simulink model "MPC_simulink"  (R2019b)
settings: Solver=VariableStepAuto  StartTime=0.0  StopTime=inf  RelTol=1e-3
InitFcn:
  | setup_NMPC
undefined symbols (not defined in the file or in its folder): MPC_func
libraries: modbusMatLib x12, simulink x7, dspstat3 x3, realtime_pacer_lib x1
settings Model: Creator=pppc  LastModifiedBy=Lenovo
settings SFSimCC: CustomCodeUndefinedFunction=UseInterfaceOnly

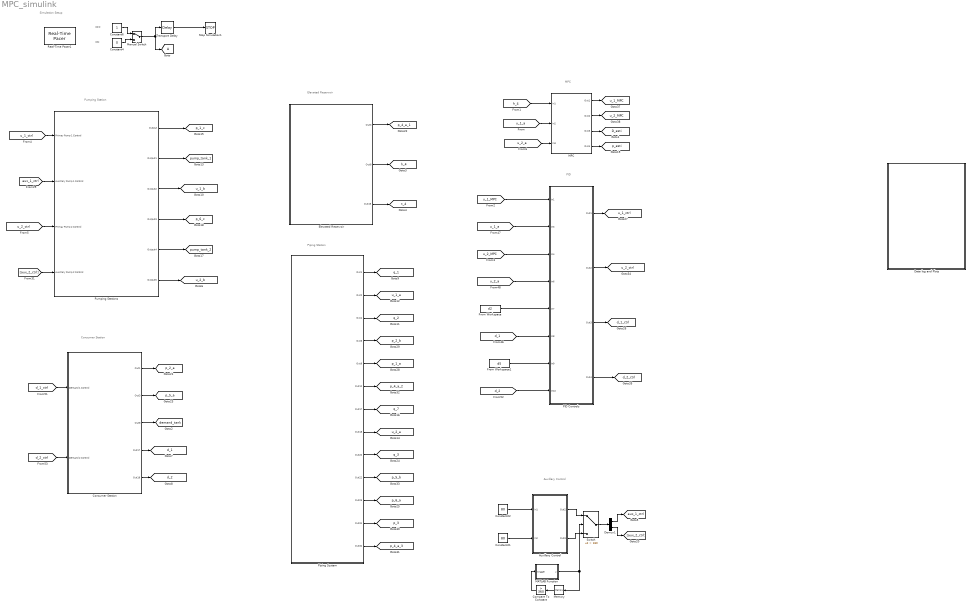
== system MPC_simulink ==
  note: Pumping Station
  note: ON
  note: Simulation Setup
  note: OFF
  note: Consumer Station
  note: Elevated Reservoir
  note: Piping Station
  note: MPC
  note: PID
  note: Auxillary Control
  Auxillary Control : Subsystem
  Compare To Constant : simulink/Logic and Bit Operations/Compare To Constant  relop=>  const=360  OutDataTypeStr=uint8
  Constant21 : Constant  Value=80
  Constant22 : Constant  Value=80
  Constant4 : Constant  Value=0
  Constant6 : Constant
  Consumer Station : Subsystem
  Data log and Plots : Subsystem
  Demux1 : Demux  Outputs=2
  "Elevated Reservoir " : Subsystem
  From Workspace : FromWorkspace  VariableName=d2  SampleTime=1
  From Workspace1 : FromWorkspace  VariableName=d5  SampleTime=1
  MATLAB Function : MATLAB Function  TreatAsAtomicUnit=on  SystemSampleTime=1
  MPC : Subsystem
  Manual Switch : ManualSwitch
  Memory : Memory
  "PID Controls " : Subsystem
  Piping System : Subsystem
  Pumping Stations : Subsystem
  Real-Time Pacer1 : realtime_pacer_lib/Real-Time Pacer  simTimePerRealTime=1
  Stop Simulation1 : Stop
  Switch : Switch  Criteria=u2 > Threshold  Threshold=180
  Transport Delay : TransportDelay  DelayTime=2
  tag scope: A=global, D_esti=global, aux_1_ctrl=global, d_1=global, d_1_ctrl=global, d_2=global, d_2_ctrl=global, demand_tank=global, h_4=global, p_1_a=global, p_1_c=global, p_2_a=global, p_2_b=global, p_3=global, p_4_a_1=global, p_4_a_2=global, p_4_a_3=global, p_5_a=global, p_5_b=global, p_6_a=global, p_6_c=global, p_esti=global, pump_tank_1=global, pump_tank_2=global, q_1=global, q_2=global, q_3=global, q_7=global, t_4=global, u_1_MPC=global, u_1_a=global, u_1_b=global, u_1_ctrl=global, u_2_MPC=global, u_2_a=global, u_2_b=global, u_2_ctrl=global
  wires:
  Manual Switch/1 -> [A], Transport Delay/1
  Constant4/1 -> Manual Switch/2
  Transport Delay/1 -> Stop Simulation1/1
  Constant6/1 -> Manual Switch/1
  [u_1_ctrl] -> Pumping Stations/1(Primay Pump 1 Control)
  [u_2_ctrl] -> Pumping Stations/3(Primay Pump 2 Control)
  [aux_2_ctrl] -> Pumping Stations/4(Auxillary Pump 2 Control)
  [aux_1_ctrl] -> Pumping Stations/2(Auxillary Pump 1 Control)
  Pumping Stations/1(Output) -> [p_1_c]
  Pumping Stations/2(Output1) -> [pump_tank_1]
  Pumping Stations/3(Output2) -> [u_1_b]
  Pumping Stations/6(Output5) -> [u_2_b]
  Pumping Stations/5(Output4) -> [pump_tank_2]
  Pumping Stations/4(Output3) -> [p_6_c]
  [d_1_ctrl] -> Consumer Station/1(Demand 1 Control)
  [d_2_ctrl] -> Consumer Station/2(Demand 2 Control)
  Consumer Station/1(Out1) -> [p_2_a]
  Consumer Station/2(Out3) -> [p_5_a]
  Consumer Station/3(Out8) -> [demand_tank]
  Consumer Station/4(Out17) -> [d_1]
  Consumer Station/5(Out19) -> [d_2]
  "Elevated Reservoir "/1(Out3) -> [p_4_a_1]
  "Elevated Reservoir "/2(Out8) -> [h_4]
  "Elevated Reservoir "/3(Out19) -> [t_4]
  Piping System/1(Out1) -> [q_1]
  Piping System/2(Out2) -> [u_1_a]
  Piping System/3(Out4) -> [q_2]
  Piping System/4(Out6) -> [p_2_b]
  Piping System/5(Out9) -> [p_1_a]
  Piping System/6(Out12) -> [p_4_a_2]
  Piping System/7(Out17) -> [q_7]
  Piping System/8(Out18) -> [u_2_a]
  Piping System/9(Out20) -> [q_3]
  Piping System/10(Out22) -> [p_5_b]
  Piping System/11(Out25) -> [p_6_a]
  Piping System/12(Out31) -> [p_3]
  Piping System/13(Out32) -> [p_4_a_3]
  [u_1_MPC] -> "PID Controls "/1(In1)
  [u_1_a] -> "PID Controls "/2(In3)
  [u_2_MPC] -> "PID Controls "/3(In4)
  [u_2_a] -> "PID Controls "/4(In6)
  From Workspace/1 -> "PID Controls "/5(In7)
  [d_1] -> "PID Controls "/6(In8)
  From Workspace1/1 -> "PID Controls "/7(In9)
  [d_2] -> "PID Controls "/8(In10)
  "PID Controls "/1(Out1) -> [u_1_ctrl]
  "PID Controls "/2(Out2) -> [u_2_ctrl]
  "PID Controls "/3(Out3) -> [d_1_ctrl]
  "PID Controls "/4(Out4) -> [d_2_ctrl]
  [h_4] -> MPC/1(In1)
  MPC/1(Out1) -> [u_1_MPC]
  MPC/2(Out2) -> [u_2_MPC]
  Constant22/1 -> Auxillary Control/1(In1)
  Constant21/1 -> Auxillary Control/2(In2)
  Demux1/1 -> [aux_1_ctrl]
  Compare To Constant/1 -> MATLAB Function/1(trigger)
  Auxillary Control/2(Out3) -> Switch/3
  Switch/1 -> Demux1/1
  Auxillary Control/1(Out2) -> Switch/1
  Demux1/2 -> [aux_2_ctrl]
  MATLAB Function/1(y) -> Switch/2, Memory/1
  Memory/1 -> Compare To Constant/1
  MPC/3(Out3) -> [D_esti]
  MPC/4(Out4) -> [p_esti]
  [u_1_a] -> MPC/2(In2)
  [u_2_a] -> MPC/3(In3)

== system MPC_simulink/Auxillary Control ==
  In1 : Inport
  In2 : Inport  Port=2
  Auxillary control : MATLAB Function  TreatAsAtomicUnit=on
  Auxillary control1 : MATLAB Function  TreatAsAtomicUnit=on
  Constant23 : Constant  Value=0
  Mux1 : Mux  Inputs=2
  Mux2 : Mux  Inputs=2
  Out2 : Outport  VectorParamsAs1DForOutWhenUnconnected=off
  Out3 : Outport  Port=2  VectorParamsAs1DForOutWhenUnconnected=off
  wires:
  Constant23/1 -> Mux2/1, Mux1/2
  Auxillary control1/1(pumpsaux) -> Mux2/2
  [demand_tank] -> Auxillary control1/1(dp)
  In2/1 -> Auxillary control1/2(u_aux)
  [demand_tank] -> Auxillary control/1(dp)
  Mux2/1 -> Out3/1
  In1/1 -> Auxillary control/2(u_aux)
  Mux1/1 -> Out2/1
  Auxillary control/1(pumpsaux) -> Mux1/1

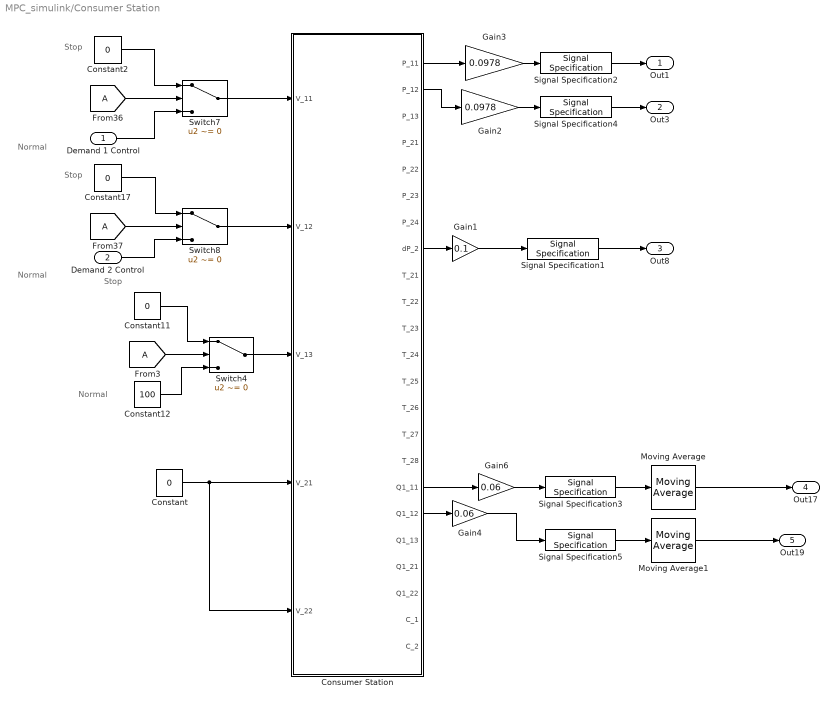
== system MPC_simulink/Consumer Station ==
  note: Normal
  note: Normal
  note: Stop
  note: Stop
  note: Normal
  note: Stop
  Demand 1 Control : Inport
  Demand 2 Control : Inport  Port=2
  Constant{,2,11,17} (4 alike) : Constant  Value=0
  Constant12 : Constant  Value=100
  Consumer Station : Subsystem
  Gain1 : Gain  Gain=0.1
  Gain2 : Gain  Gain=0.0978
  Gain3 : Gain  Gain=0.0978
  Gain4 : Gain  Gain=0.06
  Gain6 : Gain  Gain=0.06
  Moving Average : dspstat3/Moving Average  Method=Sliding window  ForgettingFactorPort=off  SpecifyWindowLength=on  WindowLength=13  ForgettingFactor=0.9  SimulateUsing=Code generation
  Moving Average1 : dspstat3/Moving Average  Method=Sliding window  ForgettingFactorPort=off  SpecifyWindowLength=on  WindowLength=13  ForgettingFactor=0.9  SimulateUsing=Code generation
  Signal Specification1 : SignalSpecification  Unit=m
  Signal Specification2 : SignalSpecification  Unit=bar
  Signal Specification3 : SignalSpecification  Unit=m^3/hr
  Signal Specification4 : SignalSpecification  Unit=bar
  Signal Specification5 : SignalSpecification  Unit=m^3/hr
  Switch4 : Switch  Criteria=u2 ~= 0
  Switch7 : Switch  Criteria=u2 ~= 0
  Switch8 : Switch  Criteria=u2 ~= 0
  Out1 : Outport  VectorParamsAs1DForOutWhenUnconnected=off
  Out3 : Outport  Port=2  VectorParamsAs1DForOutWhenUnconnected=off
  Out8 : Outport  Port=3  VectorParamsAs1DForOutWhenUnconnected=off
  Out17 : Outport  Port=4  VectorParamsAs1DForOutWhenUnconnected=off
  Out19 : Outport  Port=5  VectorParamsAs1DForOutWhenUnconnected=off
  wires:
  Constant11/1 -> Switch4/1
  Constant17/1 -> Switch8/1
  [A] -> Switch8/2
  Signal Specification1/1 -> Out8/1
  Constant12/1 -> Switch4/3
  Consumer Station/8(dP_2) -> Gain1/1
  Switch8/1 -> Consumer Station/2(V_12)
  Gain1/1 -> Signal Specification1/1
  Demand 2 Control/1 -> Switch8/3
  [A] -> Switch4/2
  Constant2/1 -> Switch7/1
  Switch4/1 -> Consumer Station/3(V_13)
  Signal Specification4/1 -> Out3/1
  Switch7/1 -> Consumer Station/1(V_11)
  Constant/1 -> Consumer Station/5(V_22), Consumer Station/4(V_21)
  [A] -> Switch7/2
  Demand 1 Control/1 -> Switch7/3
  Gain2/1 -> Signal Specification4/1
  Consumer Station/2(P_12) -> Gain2/1
  Gain3/1 -> Signal Specification2/1
  Signal Specification2/1 -> Out1/1
  Consumer Station/1(P_11) -> Gain3/1
  Signal Specification3/1 -> Moving Average/1
  Gain6/1 -> Signal Specification3/1
  Consumer Station/17(Q1_11) -> Gain6/1
  Gain4/1 -> Signal Specification5/1
  Consumer Station/18(Q1_12) -> Gain4/1
  Signal Specification5/1 -> Moving Average1/1
  Moving Average/1 -> Out17/1
  Moving Average1/1 -> Out19/1

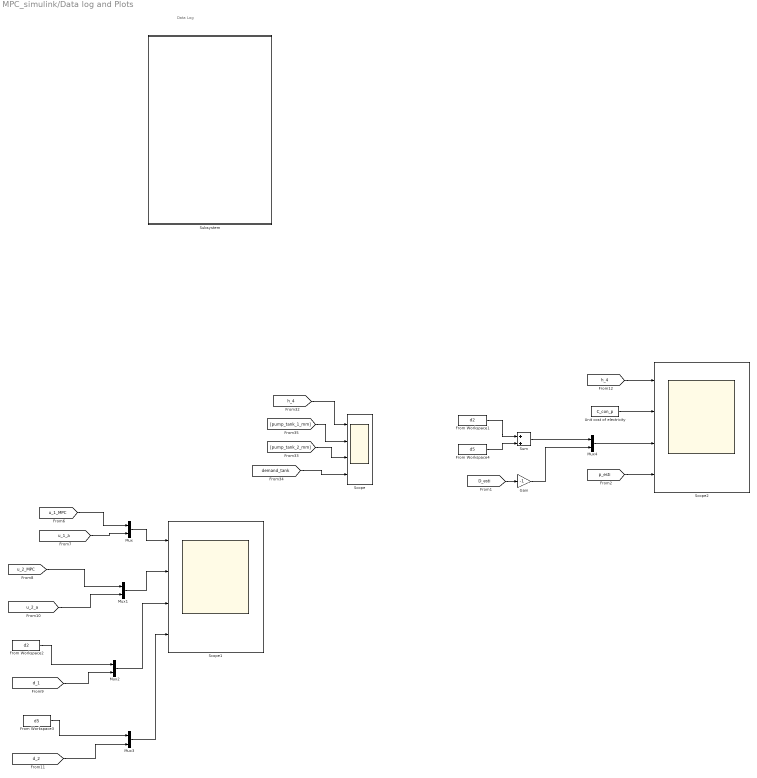
== system MPC_simulink/Data log and Plots ==
  note: Data Log
  From Workspace1 : FromWorkspace  VariableName=d2  SampleTime=1
  From Workspace2 : FromWorkspace  VariableName=d2  SampleTime=1
  From Workspace3 : FromWorkspace  VariableName=d5  SampleTime=1
  From Workspace4 : FromWorkspace  VariableName=d5  SampleTime=1
  Gain : Gain  Gain=-1
  Mux{,1..4} (5 alike) : Mux  Inputs=2
  Scope : Scope  NumInputPorts=4
  Scope1 : Scope  NumInputPorts=4
  Scope2 : Scope  NumInputPorts=4
  Subsystem : Subsystem
  Sum : Sum  Inputs=+|+
  Unit cost of electricity : FromWorkspace  VariableName=C_con_p  SampleTime=1
  wires:
  [h_4] -> Scope2/1
  Mux3/1 -> Scope1/4
  Mux2/1 -> Scope1/3
  Unit cost of electricity/1 -> Scope2/2
  [u_2_a] -> Mux1/2
  [u_1_a] -> Mux/2
  [d_1] -> Mux2/2
  From Workspace3/1 -> Mux3/1
  From Workspace2/1 -> Mux2/1
  [h_4] -> Scope/1
  [d_2] -> Mux3/2
  [u_2_MPC] -> Mux1/1
  [u_1_MPC] -> Mux/1
  Mux/1 -> Scope1/1
  Mux1/1 -> Scope1/2
  [demand_tank] -> Scope/4
  [pump_tank_2_mm] -> Scope/3
  [pump_tank_1_mm] -> Scope/2
  [p_esti] -> Scope2/4
  [D_esti] -> Gain/1
  From Workspace1/1 -> Sum/1
  Mux4/1 -> Scope2/3
  Sum/1 -> Mux4/1
  From Workspace4/1 -> Sum/2
  Gain/1 -> Mux4/2

== system MPC_simulink/Elevated Reservoir  ==
  note: Normal
  note: Stop
  Constant1 : Constant  Value=0
  Constant13 : Constant  Value=100
  Constant3 : Constant  Value=0
  Elevated Reservior : Subsystem
  Gain : Gain  Gain=0.1
  Gain3 : Gain  Gain=0.0978
  Gain6 : Gain  Gain=0.06
  Signal Specification : SignalSpecification  Unit=m
  Signal Specification3 : SignalSpecification  Unit=m^3/hr
  Signal Specification5 : SignalSpecification  Unit=bar
  Switch5 : Switch  Criteria=u2 ~= 0
  Out3 : Outport  VectorParamsAs1DForOutWhenUnconnected=off
  Out8 : Outport  Port=2  VectorParamsAs1DForOutWhenUnconnected=off
  Out19 : Outport  Port=3  VectorParamsAs1DForOutWhenUnconnected=off
  wires:
  Constant3/1 -> Elevated Reservior/5(V_22), Elevated Reservior/4(V_21), Elevated Reservior/2(V_12), Elevated Reservior/1(V_11)
  Constant13/1 -> Switch5/3
  Constant1/1 -> Switch5/1
  Elevated Reservior/8(dP_2) -> Gain/1
  Gain/1 -> Signal Specification/1
  [A] -> Switch5/2
  Switch5/1 -> Elevated Reservior/3(V_13)
  Signal Specification/1 -> Out8/1
  Signal Specification5/1 -> Out3/1
  Elevated Reservior/3(P_13) -> Gain3/1
  Gain3/1 -> Signal Specification5/1
  Gain6/1 -> Signal Specification3/1
  Elevated Reservior/19(Q1_13) -> Gain6/1
  Signal Specification3/1 -> Out19/1

== system MPC_simulink/MPC ==
  note: Pumping station 1 actual flow
  note: Level of the elevated tank
  note: Casadi NMPC and
      | Consumer demand predictor function
  note: Pumping station 2 actual flow
  note: Pumping station 1 flow command
  note: Pumping station 2 flow command
  note: Estimated level of the elevated tank
  note: Estimated consumer demand
  In1 : Inport
  In2 : Inport  Port=2
  In3 : Inport  Port=3
  Demux1 : Demux
  Gain7 : Gain  Gain=0.0978
  Interpreted MATLAB Function : MATLABFcn  MATLABFcn=MPC_func(u(1),u(2))  SampleTime=60
  Moving Average : dspstat3/Moving Average  Method=Sliding window  ForgettingFactorPort=off  SpecifyWindowLength=on  WindowLength=60  ForgettingFactor=0.9  SimulateUsing=Code generation
  Mux : Mux  Inputs=2
  Signal Specification7 : SignalSpecification  Unit=bar
  Sum : Sum  Inputs=|++
  Out1 : Outport  VectorParamsAs1DForOutWhenUnconnected=off
  Out2 : Outport  Port=2  VectorParamsAs1DForOutWhenUnconnected=off
  Out3 : Outport  Port=3  VectorParamsAs1DForOutWhenUnconnected=off
  Out4 : Outport  Port=4  VectorParamsAs1DForOutWhenUnconnected=off
  wires:
  In1/1 -> Gain7/1
  Gain7/1 -> Signal Specification7/1
  Signal Specification7/1 -> Mux/1
  Interpreted MATLAB Function/1 -> Demux1/1
  Demux1/1 -> Out1/1
  Demux1/2 -> Out2/1
  Demux1/3 -> Out3/1
  Demux1/4 -> Out4/1
  Mux/1 -> Interpreted MATLAB Function/1
  Sum/1 -> Moving Average/1
  Moving Average/1 -> Mux/2
  In2/1 -> Sum/1
  In3/1 -> Sum/2

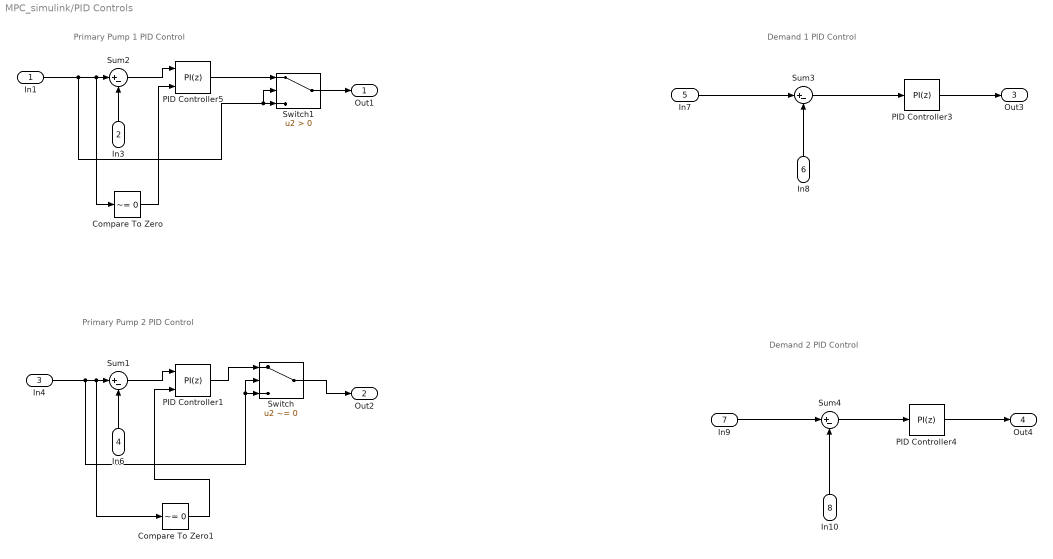
== system MPC_simulink/PID Controls  ==
  note: Primary Pump 1 PID Control
  note: Primary Pump 2 PID Control
  note: Demand 1 PID Control
  note: Demand 2 PID Control
  In1 : Inport
  In3 : Inport  Port=2
  In4 : Inport  Port=3
  In6 : Inport  Port=4
  In7 : Inport  Port=5
  In8 : Inport  Port=6
  In9 : Inport  Port=7
  In10 : Inport  Port=8
  Compare To Zero : simulink/Logic and Bit Operations/Compare To Zero  relop=~=  OutDataTypeStr=boolean
  Compare To Zero1 : simulink/Logic and Bit Operations/Compare To Zero  relop=~=  OutDataTypeStr=boolean
  PID Controller1 : simulink/Continuous/PID Controller  Controller=PI  Form=Parallel  TimeDomain=Discrete-time  SampleTime=1  IntegratorMethod=Forward Euler  FilterMethod=Forward Euler  ControllerParametersSource=internal  P=3  I=1.1  D=0  UseFilter=on  N=0  TunerSelectOption=Transfer Function Based (PID Tuner App)  InitialConditionSource=internal  InitialConditionForIntegrator=63  InitialConditionForFilter=0  DifferentiatorICPrevScaledInput=0  ExternalReset=rising  TrackingMode=off  Kt=2  LimitOutput=on  UpperSaturationLimit=95  LowerSaturationLimit=40  LinearizeAsGain=off  AntiWindupMode=clamping  Kb=1  POutMin=[]  POutMax=[]  IOutMin=[]  IOutMax=[]  DOutMin=[]  DOutMax=[]  NOutMin=[]  NOutMax=[]  SumOutMin=[]  SumOutMax=[]  SaturationOutMin=[]  SaturationOutMax=[]  PParamMin=[]  PParamMax=[]  IParamMin=[]  IParamMax=[]  DParamMin=[]  DParamMax=[]  NParamMin=[]  NParamMax=[]  KbParamMin=[]  KbParamMax=[]  KtParamMin=[]  KtParamMax=[]  KbOutMin=[]  KbOutMax=[]  KtOutMin=[]  KtOutMax=[]  IntegratorOutMin=[]  IntegratorOutMax=[]  FilterOutMin=[]  FilterOutMax=[]  SumI1OutMin=[]  SumI1OutMax=[]  SumI2OutMin=[]  SumI2OutMax=[]  SumI3OutMin=[]  SumI3OutMax=[]  SumI4OutMin=[]  SumI4OutMax=[]  SumDOutMin=[]  SumDOutMax=[]  DifferentiatorOutMin=[]  DifferentiatorOutMax=[]  FilterDiffOutCoefMin=[]  FilterDiffOutCoefMax=[]  ReciprocalOutMin=[]  ReciprocalOutMax=[]  SumDenOutMin=[]  SumDenOutMax=[]  SumNumOutMin=[]  SumNumOutMax=[]  DivideOutMin=[]  DivideOutMax=[]  IntegratorContinuousStateAttributes=''  IntegratorStateMustResolveToSignalObject=off  IntegratorRTWStateStorageClass=Auto  FilterContinuousStateAttributes=''  FilterStateMustResolveToSignalObject=off  FilterRTWStateStorageClass=Auto  ParallelPVariant=InternalParameters  IdealPVariant=Disabled  IVariant=InternalParameters  DVariant=Disabled  IntegratorVariant=Discrete  SatVariant=Enabled  AWVariant=DiscClampingParallel  PCopyVariant=Disabled  TRVariant=Disabled  FdbkBlocksVariant=Forward  IdealPFdbkVariant=Disabled  SatFdbkVariant=Disabled  DerivativeFilterVariant=Disabled  NVariant=Disabled  NCopyVariant=Disabled_SignalSpec  FilterICVariant=Disabled  IntegratorICVariant=InternalICs  ExternalResetVariant=ExternalReset  TRSumVariant=Passthrough  SumFdbkVariant=Disabled  SumVariant=Sum_PI
  PID Controller3 : simulink/Continuous/PID Controller  Controller=PI  Form=Parallel  TimeDomain=Discrete-time  SampleTime=1  IntegratorMethod=Forward Euler  FilterMethod=Forward Euler  ControllerParametersSource=internal  P=5  I=3  D=8  UseFilter=on  N=0  TunerSelectOption=Transfer Function Based (PID Tuner App)  InitialConditionSource=internal  InitialConditionForIntegrator=53  InitialConditionForFilter=0  DifferentiatorICPrevScaledInput=0  ExternalReset=none  TrackingMode=off  Kt=1  LimitOutput=on  UpperSaturationLimit=100  LowerSaturationLimit=30  LinearizeAsGain=off  AntiWindupMode=clamping  Kb=1  POutMin=[]  POutMax=[]  IOutMin=[]  IOutMax=[]  DOutMin=[]  DOutMax=[]  NOutMin=[]  NOutMax=[]  SumOutMin=[]  SumOutMax=[]  SaturationOutMin=[]  SaturationOutMax=[]  PParamMin=[]  PParamMax=[]  IParamMin=[]  IParamMax=[]  DParamMin=[]  DParamMax=[]  NParamMin=[]  NParamMax=[]  KbParamMin=[]  KbParamMax=[]  KtParamMin=[]  KtParamMax=[]  KbOutMin=[]  KbOutMax=[]  KtOutMin=[]  KtOutMax=[]  IntegratorOutMin=[]  IntegratorOutMax=[]  FilterOutMin=[]  FilterOutMax=[]  SumI1OutMin=[]  SumI1OutMax=[]  SumI2OutMin=[]  SumI2OutMax=[]  SumI3OutMin=[]  SumI3OutMax=[]  SumI4OutMin=[]  SumI4OutMax=[]  SumDOutMin=[]  SumDOutMax=[]  DifferentiatorOutMin=[]  DifferentiatorOutMax=[]  FilterDiffOutCoefMin=[]  FilterDiffOutCoefMax=[]  ReciprocalOutMin=[]  ReciprocalOutMax=[]  SumDenOutMin=[]  SumDenOutMax=[]  SumNumOutMin=[]  SumNumOutMax=[]  DivideOutMin=[]  DivideOutMax=[]  IntegratorContinuousStateAttributes=''  IntegratorStateMustResolveToSignalObject=off  IntegratorRTWStateStorageClass=Auto  FilterContinuousStateAttributes=''  FilterStateMustResolveToSignalObject=off  FilterRTWStateStorageClass=Auto  ParallelPVariant=InternalParameters  IdealPVariant=Disabled  IVariant=InternalParameters  DVariant=Disabled  IntegratorVariant=Discrete  SatVariant=Enabled  AWVariant=DiscClampingParallel  PCopyVariant=Disabled  TRVariant=Disabled  FdbkBlocksVariant=Forward  IdealPFdbkVariant=Disabled  SatFdbkVariant=Disabled  DerivativeFilterVariant=Disabled  NVariant=Disabled  NCopyVariant=Disabled_SignalSpec  FilterICVariant=Disabled  IntegratorICVariant=InternalICs  ExternalResetVariant=Disabled  TRSumVariant=Passthrough  SumFdbkVariant=Disabled  SumVariant=Sum_PI
  PID Controller4 : simulink/Continuous/PID Controller  Controller=PI  Form=Parallel  TimeDomain=Discrete-time  SampleTime=1  IntegratorMethod=Forward Euler  FilterMethod=Forward Euler  ControllerParametersSource=internal  P=5  I=2  D=8  UseFilter=on  N=0  TunerSelectOption=Transfer Function Based (PID Tuner App)  InitialConditionSource=internal  InitialConditionForIntegrator=45  InitialConditionForFilter=0  DifferentiatorICPrevScaledInput=0  ExternalReset=none  TrackingMode=off  Kt=1  LimitOutput=on  UpperSaturationLimit=100  LowerSaturationLimit=30  LinearizeAsGain=off  AntiWindupMode=clamping  Kb=1  POutMin=[]  POutMax=[]  IOutMin=[]  IOutMax=[]  DOutMin=[]  DOutMax=[]  NOutMin=[]  NOutMax=[]  SumOutMin=[]  SumOutMax=[]  SaturationOutMin=[]  SaturationOutMax=[]  PParamMin=[]  PParamMax=[]  IParamMin=[]  IParamMax=[]  DParamMin=[]  DParamMax=[]  NParamMin=[]  NParamMax=[]  KbParamMin=[]  KbParamMax=[]  KtParamMin=[]  KtParamMax=[]  KbOutMin=[]  KbOutMax=[]  KtOutMin=[]  KtOutMax=[]  IntegratorOutMin=[]  IntegratorOutMax=[]  FilterOutMin=[]  FilterOutMax=[]  SumI1OutMin=[]  SumI1OutMax=[]  SumI2OutMin=[]  SumI2OutMax=[]  SumI3OutMin=[]  SumI3OutMax=[]  SumI4OutMin=[]  SumI4OutMax=[]  SumDOutMin=[]  SumDOutMax=[]  DifferentiatorOutMin=[]  DifferentiatorOutMax=[]  FilterDiffOutCoefMin=[]  FilterDiffOutCoefMax=[]  ReciprocalOutMin=[]  ReciprocalOutMax=[]  SumDenOutMin=[]  SumDenOutMax=[]  SumNumOutMin=[]  SumNumOutMax=[]  DivideOutMin=[]  DivideOutMax=[]  IntegratorContinuousStateAttributes=''  IntegratorStateMustResolveToSignalObject=off  IntegratorRTWStateStorageClass=Auto  FilterContinuousStateAttributes=''  FilterStateMustResolveToSignalObject=off  FilterRTWStateStorageClass=Auto  ParallelPVariant=InternalParameters  IdealPVariant=Disabled  IVariant=InternalParameters  DVariant=Disabled  IntegratorVariant=Discrete  SatVariant=Enabled  AWVariant=DiscClampingParallel  PCopyVariant=Disabled  TRVariant=Disabled  FdbkBlocksVariant=Forward  IdealPFdbkVariant=Disabled  SatFdbkVariant=Disabled  DerivativeFilterVariant=Disabled  NVariant=Disabled  NCopyVariant=Disabled_SignalSpec  FilterICVariant=Disabled  IntegratorICVariant=InternalICs  ExternalResetVariant=Disabled  TRSumVariant=Passthrough  SumFdbkVariant=Disabled  SumVariant=Sum_PI
  PID Controller5 : simulink/Continuous/PID Controller  Controller=PI  Form=Parallel  TimeDomain=Discrete-time  SampleTime=1  IntegratorMethod=Forward Euler  FilterMethod=Forward Euler  ControllerParametersSource=internal  P=3  I=1.1  D=0  UseFilter=on  N=0  TunerSelectOption=Transfer Function Based (PID Tuner App)  InitialConditionSource=internal  InitialConditionForIntegrator=60  InitialConditionForFilter=0  DifferentiatorICPrevScaledInput=0  ExternalReset=rising  TrackingMode=off  Kt=1  LimitOutput=on  UpperSaturationLimit=95  LowerSaturationLimit=40  LinearizeAsGain=off  AntiWindupMode=clamping  Kb=1  POutMin=[]  POutMax=[]  IOutMin=[]  IOutMax=[]  DOutMin=[]  DOutMax=[]  NOutMin=[]  NOutMax=[]  SumOutMin=[]  SumOutMax=[]  SaturationOutMin=[]  SaturationOutMax=[]  PParamMin=[]  PParamMax=[]  IParamMin=[]  IParamMax=[]  DParamMin=[]  DParamMax=[]  NParamMin=[]  NParamMax=[]  KbParamMin=[]  KbParamMax=[]  KtParamMin=[]  KtParamMax=[]  KbOutMin=[]  KbOutMax=[]  KtOutMin=[]  KtOutMax=[]  IntegratorOutMin=[]  IntegratorOutMax=[]  FilterOutMin=[]  FilterOutMax=[]  SumI1OutMin=[]  SumI1OutMax=[]  SumI2OutMin=[]  SumI2OutMax=[]  SumI3OutMin=[]  SumI3OutMax=[]  SumI4OutMin=[]  SumI4OutMax=[]  SumDOutMin=[]  SumDOutMax=[]  DifferentiatorOutMin=[]  DifferentiatorOutMax=[]  FilterDiffOutCoefMin=[]  FilterDiffOutCoefMax=[]  ReciprocalOutMin=[]  ReciprocalOutMax=[]  SumDenOutMin=[]  SumDenOutMax=[]  SumNumOutMin=[]  SumNumOutMax=[]  DivideOutMin=[]  DivideOutMax=[]  IntegratorContinuousStateAttributes=''  IntegratorStateMustResolveToSignalObject=off  IntegratorRTWStateStorageClass=Auto  FilterContinuousStateAttributes=''  FilterStateMustResolveToSignalObject=off  FilterRTWStateStorageClass=Auto  ParallelPVariant=InternalParameters  IdealPVariant=Disabled  IVariant=InternalParameters  DVariant=Disabled  IntegratorVariant=Discrete  SatVariant=Enabled  AWVariant=DiscClampingParallel  PCopyVariant=Disabled  TRVariant=Disabled  FdbkBlocksVariant=Forward  IdealPFdbkVariant=Disabled  SatFdbkVariant=Disabled  DerivativeFilterVariant=Disabled  NVariant=Disabled  NCopyVariant=Disabled_SignalSpec  FilterICVariant=Disabled  IntegratorICVariant=InternalICs  ExternalResetVariant=ExternalReset  TRSumVariant=Passthrough  SumFdbkVariant=Disabled  SumVariant=Sum_PI
  Sum{1..4} (4 alike) : Sum  Inputs=|+-
  Switch : Switch  Criteria=u2 ~= 0
  Switch1 : Switch  Criteria=u2 > Threshold
  Out1 : Outport  VectorParamsAs1DForOutWhenUnconnected=off
  Out2 : Outport  Port=2  VectorParamsAs1DForOutWhenUnconnected=off
  Out3 : Outport  Port=3  VectorParamsAs1DForOutWhenUnconnected=off
  Out4 : Outport  Port=4  VectorParamsAs1DForOutWhenUnconnected=off
  wires:
  PID Controller1/1 -> Switch/1
  Sum1/1 -> PID Controller1/1
  In3/1 -> Sum2/2
  Sum2/1 -> PID Controller5/1
  In9/1 -> Sum4/1
  PID Controller5/1 -> Switch1/1
  In7/1 -> Sum3/1
  In6/1 -> Sum1/2
  In8/1 -> Sum3/2
  Sum3/1 -> PID Controller3/1
  In10/1 -> Sum4/2
  Sum4/1 -> PID Controller4/1
  In1/1 -> Switch1/2, Switch1/3, Compare To Zero/1, Sum2/1
  In4/1 -> Switch/2, Switch/3, Compare To Zero1/1, Sum1/1
  Switch/1 -> Out2/1
  Switch1/1 -> Out1/1
  PID Controller3/1 -> Out3/1
  PID Controller4/1 -> Out4/1
  Compare To Zero/1 -> PID Controller5/2
  Compare To Zero1/1 -> PID Controller1/2

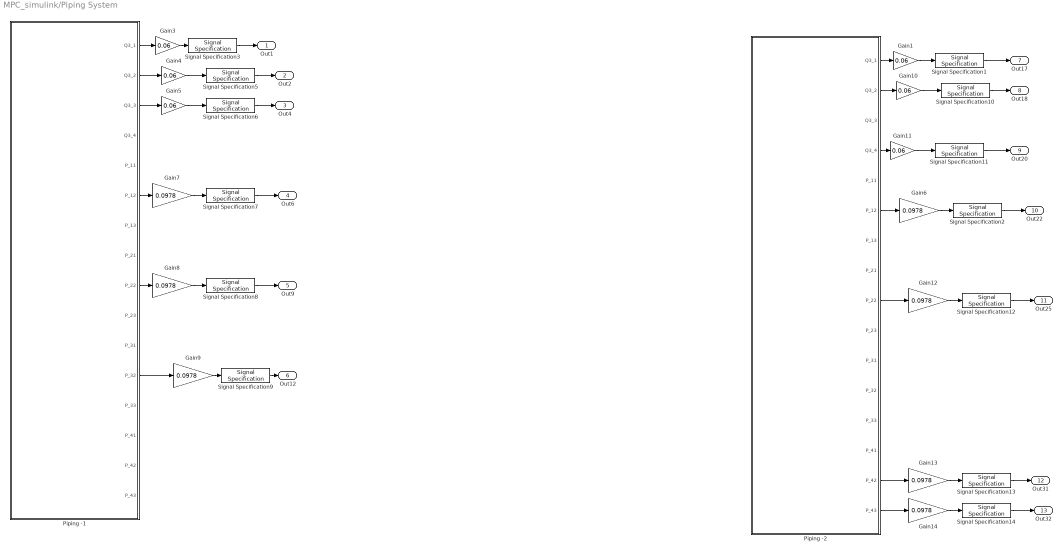
== system MPC_simulink/Piping System ==
  Gain{1,3..5,10..11} (6 alike) : Gain  Gain=0.06
  Gain{6..9,12..14} (7 alike) : Gain  Gain=0.0978
  Piping -1 : Subsystem
  Piping -2 : Subsystem
  Signal Specification{1,3,5..6,10..11} (6 alike) : SignalSpecification  Unit=m^3/hr
  Signal Specification{2,7..9,12..14} (7 alike) : SignalSpecification  Unit=bar
  Out1 : Outport  VectorParamsAs1DForOutWhenUnconnected=off
  Out2 : Outport  Port=2  VectorParamsAs1DForOutWhenUnconnected=off
  Out4 : Outport  Port=3  VectorParamsAs1DForOutWhenUnconnected=off
  Out6 : Outport  Port=4  VectorParamsAs1DForOutWhenUnconnected=off
  Out9 : Outport  Port=5  VectorParamsAs1DForOutWhenUnconnected=off
  Out12 : Outport  Port=6  VectorParamsAs1DForOutWhenUnconnected=off
  Out17 : Outport  Port=7  VectorParamsAs1DForOutWhenUnconnected=off
  Out18 : Outport  Port=8  VectorParamsAs1DForOutWhenUnconnected=off
  Out20 : Outport  Port=9  VectorParamsAs1DForOutWhenUnconnected=off
  Out22 : Outport  Port=10  VectorParamsAs1DForOutWhenUnconnected=off
  Out25 : Outport  Port=11  VectorParamsAs1DForOutWhenUnconnected=off
  Out31 : Outport  Port=12  VectorParamsAs1DForOutWhenUnconnected=off
  Out32 : Outport  Port=13  VectorParamsAs1DForOutWhenUnconnected=off
  wires:
  Piping -2/4(Q3_4) -> Gain11/1
  Piping -2/2(Q3_2) -> Gain10/1
  Piping -2/1(Q3_1) -> Gain1/1
  Signal Specification3/1 -> Out1/1
  Piping -1/1(Q3_1) -> Gain3/1
  Gain3/1 -> Signal Specification3/1
  Signal Specification5/1 -> Out2/1
  Piping -1/2(Q3_2) -> Gain4/1
  Gain4/1 -> Signal Specification5/1
  Signal Specification6/1 -> Out4/1
  Piping -1/3(Q3_3) -> Gain5/1
  Gain5/1 -> Signal Specification6/1
  Signal Specification7/1 -> Out6/1
  Piping -1/6(P_12) -> Gain7/1
  Gain7/1 -> Signal Specification7/1
  Signal Specification8/1 -> Out9/1
  Piping -1/9(P_22) -> Gain8/1
  Gain8/1 -> Signal Specification8/1
  Signal Specification9/1 -> Out12/1
  Piping -1/12(P_32) -> Gain9/1
  Gain9/1 -> Signal Specification9/1
  Signal Specification1/1 -> Out17/1
  Gain1/1 -> Signal Specification1/1
  Signal Specification10/1 -> Out18/1
  Gain10/1 -> Signal Specification10/1
  Signal Specification11/1 -> Out20/1
  Gain11/1 -> Signal Specification11/1
  Signal Specification2/1 -> Out22/1
  Piping -2/6(P_12) -> Gain6/1
  Gain6/1 -> Signal Specification2/1
  Signal Specification12/1 -> Out25/1
  Piping -2/9(P_22) -> Gain12/1
  Gain12/1 -> Signal Specification12/1
  Signal Specification13/1 -> Out31/1
  Piping -2/15(P_42) -> Gain13/1
  Gain13/1 -> Signal Specification13/1
  Signal Specification14/1 -> Out32/1
  Piping -2/16(P_43) -> Gain14/1
  Gain14/1 -> Signal Specification14/1

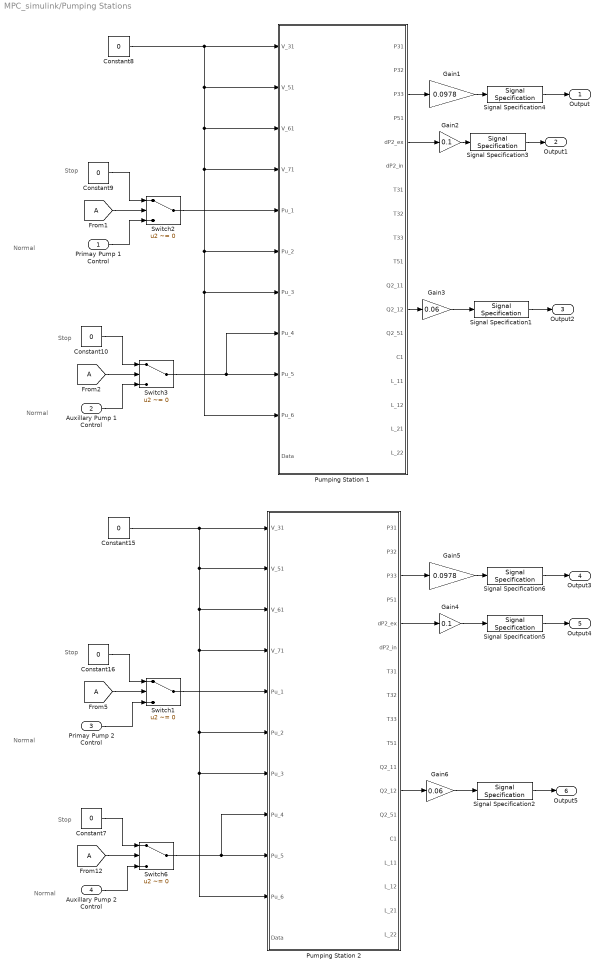
== system MPC_simulink/Pumping Stations ==
  note: Normal
  note: Stop
  note: Stop
  note: Normal
  note: Stop
  note: Normal
  note: Stop
  note: Normal
  Primay Pump 1 Control : Inport
  Auxillary Pump 1 Control : Inport  Port=2
  Primay Pump 2 Control : Inport  Port=3
  Auxillary Pump 2 Control : Inport  Port=4
  Constant{7..10,15..16} (6 alike) : Constant  Value=0
  Gain1 : Gain  Gain=0.0978
  Gain2 : Gain  Gain=0.1
  Gain3 : Gain  Gain=0.06
  Gain4 : Gain  Gain=0.1
  Gain5 : Gain  Gain=0.0978
  Gain6 : Gain  Gain=0.06
  Pumping Station 1 : Subsystem
  Pumping Station 2 : Subsystem
  Signal Specification1 : SignalSpecification  Unit=m^3/hr
  Signal Specification2 : SignalSpecification  Unit=m^3/hr
  Signal Specification3 : SignalSpecification  Unit=m
  Signal Specification4 : SignalSpecification  Unit=bar
  Signal Specification5 : SignalSpecification  Unit=m
  Signal Specification6 : SignalSpecification  Unit=bar
  Switch{1..3,6} (4 alike) : Switch  Criteria=u2 ~= 0
  Output : Outport  VectorParamsAs1DForOutWhenUnconnected=off
  Output1 : Outport  Port=2  VectorParamsAs1DForOutWhenUnconnected=off
  Output2 : Outport  Port=3  VectorParamsAs1DForOutWhenUnconnected=off
  Output3 : Outport  Port=4  VectorParamsAs1DForOutWhenUnconnected=off
  Output4 : Outport  Port=5  VectorParamsAs1DForOutWhenUnconnected=off
  Output5 : Outport  Port=6  VectorParamsAs1DForOutWhenUnconnected=off
  wires:
  Constant16/1 -> Switch1/1
  [A] -> Switch1/2
  Primay Pump 1 Control/1 -> Switch2/3
  Pumping Station 2/3(P33) -> Gain5/1
  Signal Specification3/1 -> Output1/1
  Gain1/1 -> Signal Specification4/1
  Primay Pump 2 Control/1 -> Switch1/3
  Pumping Station 1/5(dP2_ex) -> Gain2/1
  Pumping Station 2/5(dP2_ex) -> Gain4/1
  Switch6/1 -> Pumping Station 2/8(Pu_4), Pumping Station 2/9(Pu_5)
  Gain2/1 -> Signal Specification3/1
  [A] -> Switch2/2
  Switch3/1 -> Pumping Station 1/8(Pu_4), Pumping Station 1/9(Pu_5)
  Switch2/1 -> Pumping Station 1/5(Pu_1)
  Signal Specification6/1 -> Output3/1
  Auxillary Pump 1 Control/1 -> Switch3/3
  [A] -> Switch3/2
  Constant9/1 -> Switch2/1
  Signal Specification4/1 -> Output/1
  Signal Specification5/1 -> Output4/1
  Gain5/1 -> Signal Specification6/1
  Constant7/1 -> Switch6/1
  Gain4/1 -> Signal Specification5/1
  Switch1/1 -> Pumping Station 2/5(Pu_1)
  Constant10/1 -> Switch3/1
  Auxillary Pump 2 Control/1 -> Switch6/3
  Pumping Station 1/3(P33) -> Gain1/1
  [A] -> Switch6/2
  Signal Specification1/1 -> Output2/1
  Pumping Station 1/12(Q2_12) -> Gain3/1
  Gain3/1 -> Signal Specification1/1
  Signal Specification2/1 -> Output5/1
  Pumping Station 2/12(Q2_12) -> Gain6/1
  Gain6/1 -> Signal Specification2/1
  Constant15/1 -> Pumping Station 2/6(Pu_2), Pumping Station 2/10(Pu_6), Pumping Station 2/7(Pu_3), Pumping Station 2/4(V_71), Pumping Station 2/3(V_61), Pumping Station 2/2(V_51), Pumping Station 2/1(V_31)
  Constant8/1 -> Pumping Station 1/10(Pu_6), Pumping Station 1/7(Pu_3), Pumping Station 1/6(Pu_2), Pumping Station 1/4(V_71), Pumping Station 1/3(V_61), Pumping Station 1/2(V_51), Pumping Station 1/1(V_31)

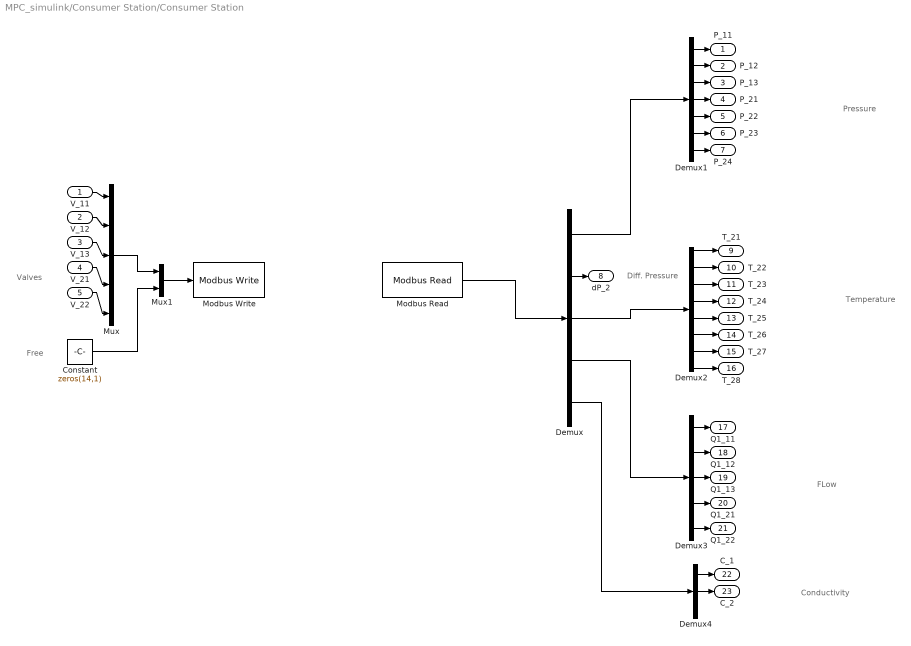
== system MPC_simulink/Consumer Station/Consumer Station ==
  note: Pressure
  note: Temperature
  note: FLow
  note: Conductivity
  note: Valves
  note: Diff. Pressure
  note: Free
  V_11 : Inport
  V_12 : Inport  Port=2
  V_13 : Inport  Port=3
  V_21 : Inport  Port=4
  V_22 : Inport  Port=5
  Constant : Constant  Value=zeros(14,1)
  Demux : Demux  Outputs=[7 1 8 5 3]
  Demux1 : Demux  Outputs=7
  Demux2 : Demux  Outputs=8
  Demux3 : Demux  Outputs=5
  Demux4 : Demux  Outputs=3
  Modbus Read : modbusMatLib/Modbus Read  registry=0  ipAddress='192.168.100.31'  port=502
  Modbus Write : modbusMatLib/Modbus Write  registry=001  port=502  ipAddress='192.168.100.31'
  Mux : Mux  Inputs=5
  Mux1 : Mux  Inputs=2
  P_11 : Outport  VectorParamsAs1DForOutWhenUnconnected=off
  P_12 : Outport  Port=2  VectorParamsAs1DForOutWhenUnconnected=off
  P_13 : Outport  Port=3  VectorParamsAs1DForOutWhenUnconnected=off
  P_21 : Outport  Port=4  VectorParamsAs1DForOutWhenUnconnected=off
  P_22 : Outport  Port=5  VectorParamsAs1DForOutWhenUnconnected=off
  P_23 : Outport  Port=6  VectorParamsAs1DForOutWhenUnconnected=off
  P_24 : Outport  Port=7  VectorParamsAs1DForOutWhenUnconnected=off
  dP_2 : Outport  Port=8  VectorParamsAs1DForOutWhenUnconnected=off
  T_21 : Outport  Port=9  VectorParamsAs1DForOutWhenUnconnected=off
  T_22 : Outport  Port=10  VectorParamsAs1DForOutWhenUnconnected=off
  T_23 : Outport  Port=11  VectorParamsAs1DForOutWhenUnconnected=off
  T_24 : Outport  Port=12  VectorParamsAs1DForOutWhenUnconnected=off
  T_25 : Outport  Port=13  VectorParamsAs1DForOutWhenUnconnected=off
  T_26 : Outport  Port=14  VectorParamsAs1DForOutWhenUnconnected=off
  T_27 : Outport  Port=15  VectorParamsAs1DForOutWhenUnconnected=off
  T_28 : Outport  Port=16  VectorParamsAs1DForOutWhenUnconnected=off
  Q1_11 : Outport  Port=17  VectorParamsAs1DForOutWhenUnconnected=off
  Q1_12 : Outport  Port=18  VectorParamsAs1DForOutWhenUnconnected=off
  Q1_13 : Outport  Port=19  VectorParamsAs1DForOutWhenUnconnected=off
  Q1_21 : Outport  Port=20  VectorParamsAs1DForOutWhenUnconnected=off
  Q1_22 : Outport  Port=21  VectorParamsAs1DForOutWhenUnconnected=off
  C_1 : Outport  Port=22  VectorParamsAs1DForOutWhenUnconnected=off
  C_2 : Outport  Port=23  VectorParamsAs1DForOutWhenUnconnected=off
  wires:
  Mux/1 -> Mux1/1
  Mux1/1 -> Modbus Write/1
  Constant/1 -> Mux1/2
  Demux1/5 -> P_22/1
  V_12/1 -> Mux/2
  Demux1/6 -> P_23/1
  Demux1/3 -> P_13/1
  Demux1/4 -> P_21/1
  V_13/1 -> Mux/3
  Demux3/2 -> Q1_12/1
  Demux3/5 -> Q1_22/1
  Demux/2 -> dP_2/1
  Demux3/1 -> Q1_11/1
  Demux1/2 -> P_12/1
  Demux2/5 -> T_25/1
  Demux4/1 -> C_1/1
  V_21/1 -> Mux/4
  Demux3/3 -> Q1_13/1
  Demux1/1 -> P_11/1
  Demux3/4 -> Q1_21/1
  V_11/1 -> Mux/1
  Demux2/4 -> T_24/1
  Demux2/3 -> T_23/1
  Demux2/2 -> T_22/1
  Demux2/1 -> T_21/1
  Demux1/7 -> P_24/1
  V_22/1 -> Mux/5
  Demux2/7 -> T_27/1
  Demux/5 -> Demux4/1
  Demux/1 -> Demux1/1
  Demux2/8 -> T_28/1
  Demux4/2 -> C_2/1
  Demux/3 -> Demux2/1
  Demux/4 -> Demux3/1
  Modbus Read/1 -> Demux/1
  Demux2/6 -> T_26/1

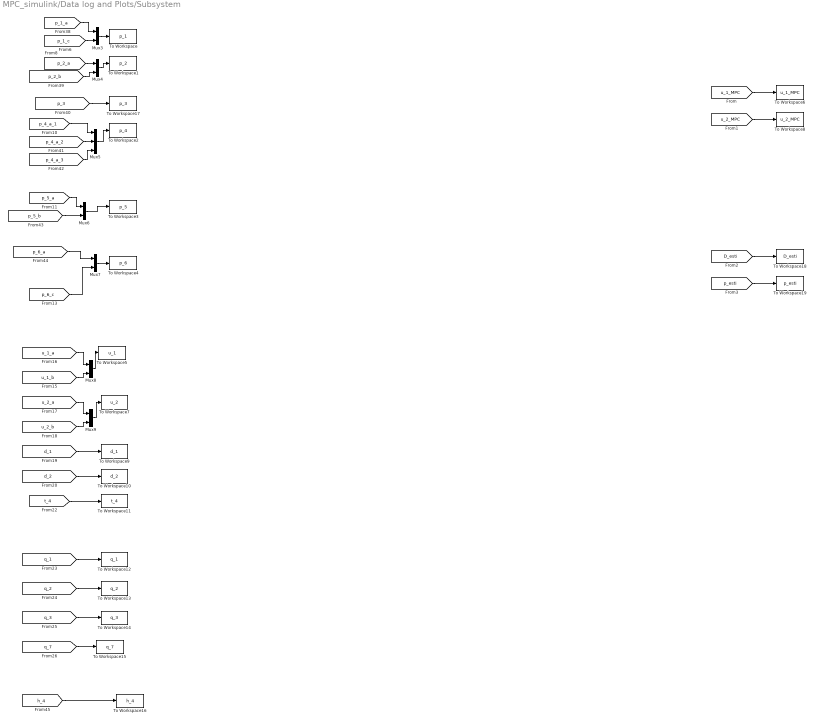
== system MPC_simulink/Data log and Plots/Subsystem ==
  Mux{3..4,6..9} (6 alike) : Mux  Inputs=2
  Mux5 : Mux  Inputs=3
  To Workspace : ToWorkspace  VariableName=p_1  SampleTime=1
      settings: Save2DSignal=2-D array (concatenate along first dimension)
  To Workspace1 : ToWorkspace  VariableName=p_2  SampleTime=1
      settings: Save2DSignal=2-D array (concatenate along first dimension)
  To Workspace10 : ToWorkspace  VariableName=d_2  SampleTime=1
      settings: Save2DSignal=2-D array (concatenate along first dimension)
  To Workspace11 : ToWorkspace  VariableName=t_4  SampleTime=1
      settings: Save2DSignal=2-D array (concatenate along first dimension)
  To Workspace12 : ToWorkspace  VariableName=q_1  SampleTime=1
      settings: Save2DSignal=2-D array (concatenate along first dimension)
  To Workspace13 : ToWorkspace  VariableName=q_2  SampleTime=1
      settings: Save2DSignal=2-D array (concatenate along first dimension)
  To Workspace14 : ToWorkspace  VariableName=q_3  SampleTime=1
      settings: Save2DSignal=2-D array (concatenate along first dimension)
  To Workspace15 : ToWorkspace  VariableName=q_7  SampleTime=1
      settings: Save2DSignal=2-D array (concatenate along first dimension)
  To Workspace16 : ToWorkspace  VariableName=h_4  SampleTime=1
      settings: Save2DSignal=2-D array (concatenate along first dimension)
  To Workspace17 : ToWorkspace  VariableName=p_3  SampleTime=1
      settings: Save2DSignal=2-D array (concatenate along first dimension)
  To Workspace18 : ToWorkspace  VariableName=D_esti  SampleTime=1
      settings: Save2DSignal=2-D array (concatenate along first dimension)
  To Workspace19 : ToWorkspace  VariableName=p_esti  SampleTime=1
      settings: Save2DSignal=2-D array (concatenate along first dimension)
  To Workspace2 : ToWorkspace  VariableName=p_4  SampleTime=1
      settings: Save2DSignal=2-D array (concatenate along first dimension)
  To Workspace3 : ToWorkspace  VariableName=p_5  SampleTime=1
      settings: Save2DSignal=2-D array (concatenate along first dimension)
  To Workspace4 : ToWorkspace  VariableName=p_6  SampleTime=1
      settings: Save2DSignal=2-D array (concatenate along first dimension)
  To Workspace5 : ToWorkspace  VariableName=u_1  SampleTime=1
      settings: Save2DSignal=2-D array (concatenate along first dimension)
  To Workspace6 : ToWorkspace  VariableName=u_1_MPC  SampleTime=1
      settings: Save2DSignal=2-D array (concatenate along first dimension)
  To Workspace7 : ToWorkspace  VariableName=u_2  SampleTime=1
      settings: Save2DSignal=2-D array (concatenate along first dimension)
  To Workspace8 : ToWorkspace  VariableName=u_2_MPC  SampleTime=1
      settings: Save2DSignal=2-D array (concatenate along first dimension)
  To Workspace9 : ToWorkspace  VariableName=d_1  SampleTime=1
      settings: Save2DSignal=2-D array (concatenate along first dimension)
  wires:
  [p_1_c] -> Mux3/2
  [p_2_a] -> Mux4/1
  [t_4] -> To Workspace11/1
  [p_1_a] -> Mux3/1
  [p_4_a_3] -> Mux5/3
  [h_4] -> To Workspace16/1
  Mux9/1 -> To Workspace7/1
  Mux6/1 -> To Workspace3/1
  [p_6_a] -> Mux7/1
  [d_1] -> To Workspace9/1
  [p_6_c] -> Mux7/2
  [p_4_a_2] -> Mux5/2
  Mux8/1 -> To Workspace5/1
  Mux3/1 -> To Workspace/1
  [q_3] -> To Workspace14/1
  Mux4/1 -> To Workspace1/1
  [d_2] -> To Workspace10/1
  [p_5_a] -> Mux6/1
  [q_2] -> To Workspace13/1
  Mux7/1 -> To Workspace4/1
  [u_2_b] -> Mux9/2
  [u_1_b] -> Mux8/2
  Mux5/1 -> To Workspace2/1
  [p_2_b] -> Mux4/2
  [u_2_a] -> Mux9/1
  [q_7] -> To Workspace15/1
  [p_4_a_1] -> Mux5/1
  [q_1] -> To Workspace12/1
  [u_1_a] -> Mux8/1
  [p_3] -> To Workspace17/1
  [p_5_b] -> Mux6/2
  [u_1_MPC] -> To Workspace6/1
  [u_2_MPC] -> To Workspace8/1
  [p_esti] -> To Workspace19/1
  [D_esti] -> To Workspace18/1

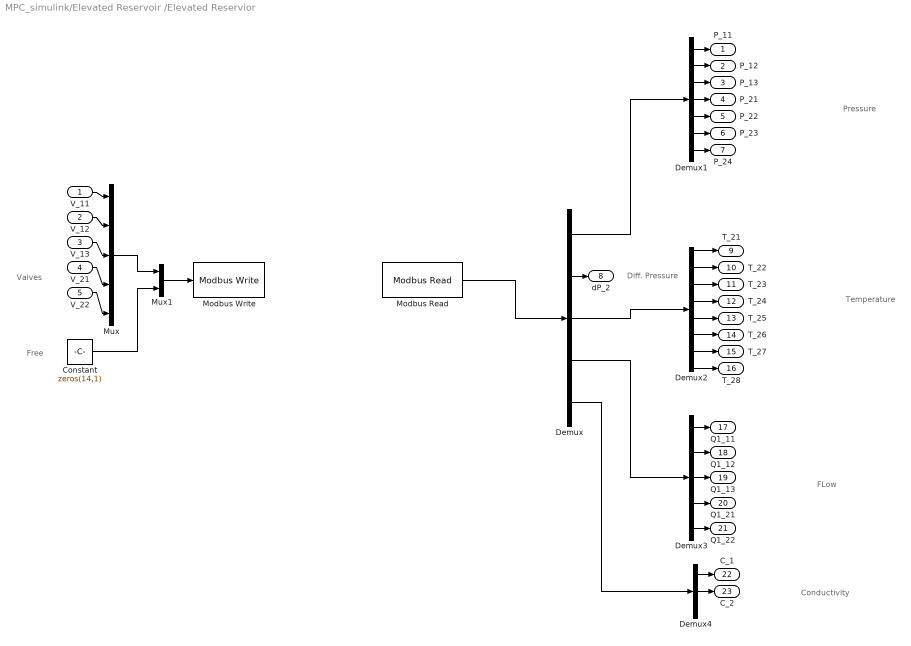
== system MPC_simulink/Elevated Reservoir /Elevated Reservior ==
  note: Pressure
  note: Temperature
  note: FLow
  note: Conductivity
  note: Valves
  note: Diff. Pressure
  note: Free
  V_11 : Inport
  V_12 : Inport  Port=2
  V_13 : Inport  Port=3
  V_21 : Inport  Port=4
  V_22 : Inport  Port=5
  Constant : Constant  Value=zeros(14,1)
  Demux : Demux  Outputs=[7 1 8 5 3]
  Demux1 : Demux  Outputs=7
  Demux2 : Demux  Outputs=8
  Demux3 : Demux  Outputs=5
  Demux4 : Demux  Outputs=3
  Modbus Read : modbusMatLib/Modbus Read  registry=0  ipAddress='192.168.100.30'  port=502
  Modbus Write : modbusMatLib/Modbus Write  registry=001  port=502  ipAddress='192.168.100.30'
  Mux : Mux  Inputs=5
  Mux1 : Mux  Inputs=2
  P_11 : Outport  VectorParamsAs1DForOutWhenUnconnected=off
  P_12 : Outport  Port=2  VectorParamsAs1DForOutWhenUnconnected=off
  P_13 : Outport  Port=3  VectorParamsAs1DForOutWhenUnconnected=off
  P_21 : Outport  Port=4  VectorParamsAs1DForOutWhenUnconnected=off
  P_22 : Outport  Port=5  VectorParamsAs1DForOutWhenUnconnected=off
  P_23 : Outport  Port=6  VectorParamsAs1DForOutWhenUnconnected=off
  P_24 : Outport  Port=7  VectorParamsAs1DForOutWhenUnconnected=off
  dP_2 : Outport  Port=8  VectorParamsAs1DForOutWhenUnconnected=off
  T_21 : Outport  Port=9  VectorParamsAs1DForOutWhenUnconnected=off
  T_22 : Outport  Port=10  VectorParamsAs1DForOutWhenUnconnected=off
  T_23 : Outport  Port=11  VectorParamsAs1DForOutWhenUnconnected=off
  T_24 : Outport  Port=12  VectorParamsAs1DForOutWhenUnconnected=off
  T_25 : Outport  Port=13  VectorParamsAs1DForOutWhenUnconnected=off
  T_26 : Outport  Port=14  VectorParamsAs1DForOutWhenUnconnected=off
  T_27 : Outport  Port=15  VectorParamsAs1DForOutWhenUnconnected=off
  T_28 : Outport  Port=16  VectorParamsAs1DForOutWhenUnconnected=off
  Q1_11 : Outport  Port=17  VectorParamsAs1DForOutWhenUnconnected=off
  Q1_12 : Outport  Port=18  VectorParamsAs1DForOutWhenUnconnected=off
  Q1_13 : Outport  Port=19  VectorParamsAs1DForOutWhenUnconnected=off
  Q1_21 : Outport  Port=20  VectorParamsAs1DForOutWhenUnconnected=off
  Q1_22 : Outport  Port=21  VectorParamsAs1DForOutWhenUnconnected=off
  C_1 : Outport  Port=22  VectorParamsAs1DForOutWhenUnconnected=off
  C_2 : Outport  Port=23  VectorParamsAs1DForOutWhenUnconnected=off
  wires:
  Mux/1 -> Mux1/1
  Mux1/1 -> Modbus Write/1
  Constant/1 -> Mux1/2
  Demux1/5 -> P_22/1
  V_12/1 -> Mux/2
  Demux1/6 -> P_23/1
  Demux1/3 -> P_13/1
  Demux1/4 -> P_21/1
  V_13/1 -> Mux/3
  Demux3/2 -> Q1_12/1
  Demux3/5 -> Q1_22/1
  Demux/2 -> dP_2/1
  Demux3/1 -> Q1_11/1
  Demux1/2 -> P_12/1
  Demux2/5 -> T_25/1
  Demux4/1 -> C_1/1
  V_21/1 -> Mux/4
  Demux3/3 -> Q1_13/1
  Demux1/1 -> P_11/1
  Demux3/4 -> Q1_21/1
  V_11/1 -> Mux/1
  Demux2/4 -> T_24/1
  Demux2/3 -> T_23/1
  Demux2/2 -> T_22/1
  Demux2/1 -> T_21/1
  Demux1/7 -> P_24/1
  V_22/1 -> Mux/5
  Demux2/7 -> T_27/1
  Demux/5 -> Demux4/1
  Demux/1 -> Demux1/1
  Demux2/8 -> T_28/1
  Demux4/2 -> C_2/1
  Demux/3 -> Demux2/1
  Demux/4 -> Demux3/1
  Modbus Read/1 -> Demux/1
  Demux2/6 -> T_26/1

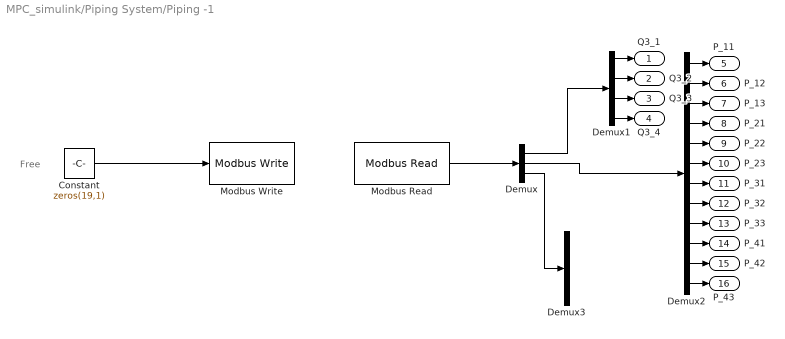
== system MPC_simulink/Piping System/Piping -1 ==
  note: Free
  Constant : Constant  Value=zeros(19,1)
  Demux : Demux  Outputs=[4 12 8]
  Demux1 : Demux
  Demux2 : Demux  Outputs=12
  Demux3 : Demux
  Modbus Read : modbusMatLib/Modbus Read  registry=0  ipAddress='192.168.100.20'  port=502
  Modbus Write : modbusMatLib/Modbus Write  registry=001  port=502  ipAddress='192.168.100.20'
  Q3_1 : Outport  VectorParamsAs1DForOutWhenUnconnected=off
  Q3_2 : Outport  Port=2  VectorParamsAs1DForOutWhenUnconnected=off
  Q3_3 : Outport  Port=3  VectorParamsAs1DForOutWhenUnconnected=off
  Q3_4 : Outport  Port=4  VectorParamsAs1DForOutWhenUnconnected=off
  P_11 : Outport  Port=5  VectorParamsAs1DForOutWhenUnconnected=off
  P_12 : Outport  Port=6  VectorParamsAs1DForOutWhenUnconnected=off
  P_13 : Outport  Port=7  VectorParamsAs1DForOutWhenUnconnected=off
  P_21 : Outport  Port=8  VectorParamsAs1DForOutWhenUnconnected=off
  P_22 : Outport  Port=9  VectorParamsAs1DForOutWhenUnconnected=off
  P_23 : Outport  Port=10  VectorParamsAs1DForOutWhenUnconnected=off
  P_31 : Outport  Port=11  VectorParamsAs1DForOutWhenUnconnected=off
  P_32 : Outport  Port=12  VectorParamsAs1DForOutWhenUnconnected=off
  P_33 : Outport  Port=13  VectorParamsAs1DForOutWhenUnconnected=off
  P_41 : Outport  Port=14  VectorParamsAs1DForOutWhenUnconnected=off
  P_42 : Outport  Port=15  VectorParamsAs1DForOutWhenUnconnected=off
  P_43 : Outport  Port=16  VectorParamsAs1DForOutWhenUnconnected=off
  wires:
  Demux1/4 -> Q3_4/1
  Demux1/2 -> Q3_2/1
  Demux1/1 -> Q3_1/1
  Demux1/3 -> Q3_3/1
  Demux/1 -> Demux1/1
  Modbus Read/1 -> Demux/1
  Constant/1 -> Modbus Write/1
  Demux/2 -> Demux2/1
  Demux/3 -> Demux3/1
  Demux2/1 -> P_11/1
  Demux2/2 -> P_12/1
  Demux2/3 -> P_13/1
  Demux2/4 -> P_21/1
  Demux2/5 -> P_22/1
  Demux2/6 -> P_23/1
  Demux2/7 -> P_31/1
  Demux2/8 -> P_32/1
  Demux2/9 -> P_33/1
  Demux2/10 -> P_41/1
  Demux2/11 -> P_42/1
  Demux2/12 -> P_43/1

== system MPC_simulink/Piping System/Piping -2 ==
  note: Free
  Constant : Constant  Value=zeros(19,1)
  Demux : Demux  Outputs=[4 12 8]
  Demux1 : Demux
  Demux2 : Demux  Outputs=12
  Demux3 : Demux
  Modbus Read : modbusMatLib/Modbus Read  registry=0  ipAddress='192.168.100.21'  port=502
  Modbus Write : modbusMatLib/Modbus Write  registry=001  port=502  ipAddress='192.168.100.21'
  Q3_1 : Outport  VectorParamsAs1DForOutWhenUnconnected=off
  Q3_2 : Outport  Port=2  VectorParamsAs1DForOutWhenUnconnected=off
  Q3_3 : Outport  Port=3  VectorParamsAs1DForOutWhenUnconnected=off
  Q3_4 : Outport  Port=4  VectorParamsAs1DForOutWhenUnconnected=off
  P_11 : Outport  Port=5  VectorParamsAs1DForOutWhenUnconnected=off
  P_12 : Outport  Port=6  VectorParamsAs1DForOutWhenUnconnected=off
  P_13 : Outport  Port=7  VectorParamsAs1DForOutWhenUnconnected=off
  P_21 : Outport  Port=8  VectorParamsAs1DForOutWhenUnconnected=off
  P_22 : Outport  Port=9  VectorParamsAs1DForOutWhenUnconnected=off
  P_23 : Outport  Port=10  VectorParamsAs1DForOutWhenUnconnected=off
  P_31 : Outport  Port=11  VectorParamsAs1DForOutWhenUnconnected=off
  P_32 : Outport  Port=12  VectorParamsAs1DForOutWhenUnconnected=off
  P_33 : Outport  Port=13  VectorParamsAs1DForOutWhenUnconnected=off
  P_41 : Outport  Port=14  VectorParamsAs1DForOutWhenUnconnected=off
  P_42 : Outport  Port=15  VectorParamsAs1DForOutWhenUnconnected=off
  P_43 : Outport  Port=16  VectorParamsAs1DForOutWhenUnconnected=off
  wires:
  Demux1/4 -> Q3_4/1
  Demux1/2 -> Q3_2/1
  Demux1/1 -> Q3_1/1
  Demux1/3 -> Q3_3/1
  Demux/1 -> Demux1/1
  Modbus Read/1 -> Demux/1
  Constant/1 -> Modbus Write/1
  Demux/2 -> Demux2/1
  Demux/3 -> Demux3/1
  Demux2/1 -> P_11/1
  Demux2/2 -> P_12/1
  Demux2/3 -> P_13/1
  Demux2/4 -> P_21/1
  Demux2/5 -> P_22/1
  Demux2/6 -> P_23/1
  Demux2/7 -> P_31/1
  Demux2/8 -> P_32/1
  Demux2/9 -> P_33/1
  Demux2/10 -> P_41/1
  Demux2/11 -> P_42/1
  Demux2/12 -> P_43/1

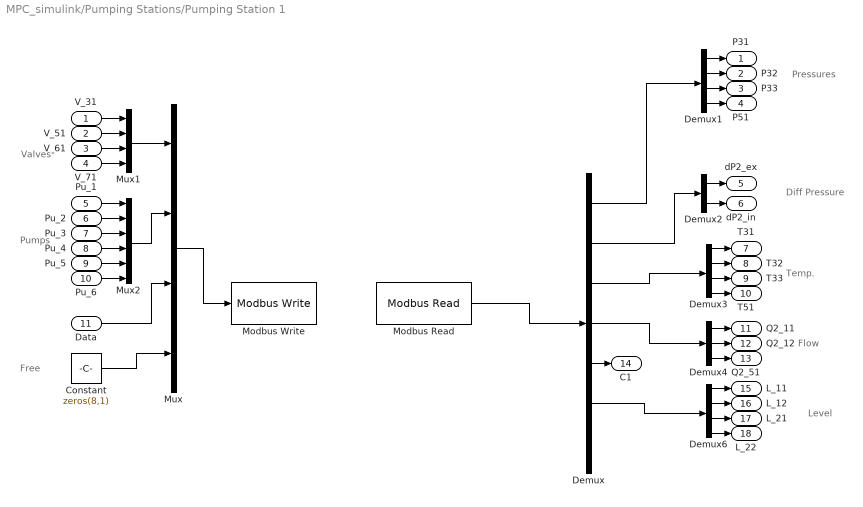
== system MPC_simulink/Pumping Stations/Pumping Station 1 ==
  note: Free
  note: Pumps
  note: Valves
  note: Flow
  note: Temp.
  note: Diff Pressure
  note: Pressures
  note: Level
  V_31 : Inport
  V_51 : Inport  Port=2
  V_61 : Inport  Port=3
  V_71 : Inport  Port=4
  Pu_1 : Inport  Port=5
  Pu_2 : Inport  Port=6
  Pu_3 : Inport  Port=7
  Pu_4 : Inport  Port=8
  Pu_5 : Inport  Port=9
  Pu_6 : Inport  Port=10
  Data : Inport  Port=11
  Constant : Constant  Value=zeros(8,1)
  Demux : Demux  Outputs=[4 2 4 3 1 4 6]
  Demux1 : Demux
  Demux2 : Demux  Outputs=2
  Demux3 : Demux
  Demux4 : Demux  Outputs=3
  Demux6 : Demux
  Modbus Read : modbusMatLib/Modbus Read  registry=0  ipAddress='192.168.100.41'  port=502
  Modbus Write : modbusMatLib/Modbus Write  registry=001  port=502  ipAddress='192.168.100.41'
  Mux : Mux
  Mux1 : Mux
  Mux2 : Mux  Inputs=6
  P31 : Outport  VectorParamsAs1DForOutWhenUnconnected=off
  P32 : Outport  Port=2  VectorParamsAs1DForOutWhenUnconnected=off
  P33 : Outport  Port=3  VectorParamsAs1DForOutWhenUnconnected=off
  P51 : Outport  Port=4  VectorParamsAs1DForOutWhenUnconnected=off
  dP2_ex : Outport  Port=5  VectorParamsAs1DForOutWhenUnconnected=off
  dP2_in : Outport  Port=6  VectorParamsAs1DForOutWhenUnconnected=off
  T31 : Outport  Port=7  VectorParamsAs1DForOutWhenUnconnected=off
  T32 : Outport  Port=8  VectorParamsAs1DForOutWhenUnconnected=off
  T33 : Outport  Port=9  VectorParamsAs1DForOutWhenUnconnected=off
  T51 : Outport  Port=10  VectorParamsAs1DForOutWhenUnconnected=off
  Q2_11 : Outport  Port=11  VectorParamsAs1DForOutWhenUnconnected=off
  Q2_12 : Outport  Port=12  VectorParamsAs1DForOutWhenUnconnected=off
  Q2_51 : Outport  Port=13  VectorParamsAs1DForOutWhenUnconnected=off
  C1 : Outport  Port=14  VectorParamsAs1DForOutWhenUnconnected=off
  L_11 : Outport  Port=15  VectorParamsAs1DForOutWhenUnconnected=off
  L_12 : Outport  Port=16  VectorParamsAs1DForOutWhenUnconnected=off
  L_21 : Outport  Port=17  VectorParamsAs1DForOutWhenUnconnected=off
  L_22 : Outport  Port=18  VectorParamsAs1DForOutWhenUnconnected=off
  wires:
  Demux4/1 -> Q2_11/1
  Demux/2 -> Demux2/1
  Demux/4 -> Demux4/1
  Demux2/1 -> dP2_ex/1
  Demux/3 -> Demux3/1
  Demux/6 -> Demux6/1
  Demux/1 -> Demux1/1
  Demux3/4 -> T51/1
  Demux1/4 -> P51/1
  Demux3/2 -> T32/1
  Modbus Read/1 -> Demux/1
  Demux6/1 -> L_11/1
  Demux6/2 -> L_12/1
  Demux4/3 -> Q2_51/1
  Demux4/2 -> Q2_12/1
  Demux6/3 -> L_21/1
  Demux6/4 -> L_22/1
  Demux3/3 -> T33/1
  Demux1/1 -> P31/1
  Demux1/2 -> P32/1
  Demux/5 -> C1/1
  Demux1/3 -> P33/1
  Demux2/2 -> dP2_in/1
  Demux3/1 -> T31/1
  Mux/1 -> Modbus Write/1
  Mux1/1 -> Mux/1
  V_31/1 -> Mux1/1
  V_51/1 -> Mux1/2
  V_61/1 -> Mux1/3
  V_71/1 -> Mux1/4
  Pu_4/1 -> Mux2/4
  Pu_3/1 -> Mux2/3
  Pu_1/1 -> Mux2/1
  Pu_2/1 -> Mux2/2
  Mux2/1 -> Mux/2
  Pu_5/1 -> Mux2/5
  Pu_6/1 -> Mux2/6
  Data/1 -> Mux/3
  Constant/1 -> Mux/4

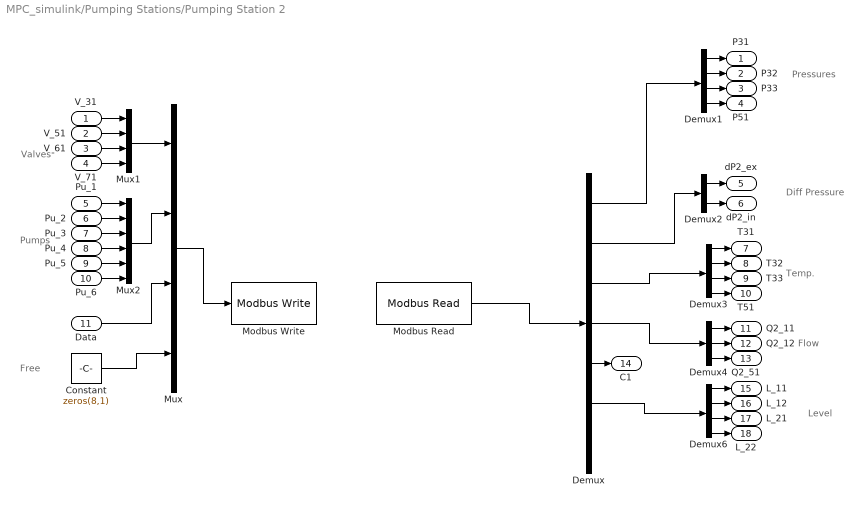
== system MPC_simulink/Pumping Stations/Pumping Station 2 ==
  note: Free
  note: Pumps
  note: Valves
  note: Flow
  note: Temp.
  note: Diff Pressure
  note: Pressures
  note: Level
  V_31 : Inport
  V_51 : Inport  Port=2
  V_61 : Inport  Port=3
  V_71 : Inport  Port=4
  Pu_1 : Inport  Port=5
  Pu_2 : Inport  Port=6
  Pu_3 : Inport  Port=7
  Pu_4 : Inport  Port=8
  Pu_5 : Inport  Port=9
  Pu_6 : Inport  Port=10
  Data : Inport  Port=11
  Constant : Constant  Value=zeros(8,1)
  Demux : Demux  Outputs=[4 2 4 3 1 4 6]
  Demux1 : Demux
  Demux2 : Demux  Outputs=2
  Demux3 : Demux
  Demux4 : Demux  Outputs=3
  Demux6 : Demux
  Modbus Read : modbusMatLib/Modbus Read  registry=0  ipAddress='192.168.100.42'  port=502
  Modbus Write : modbusMatLib/Modbus Write  registry=001  port=502  ipAddress='192.168.100.42'
  Mux : Mux
  Mux1 : Mux
  Mux2 : Mux  Inputs=6
  P31 : Outport  VectorParamsAs1DForOutWhenUnconnected=off
  P32 : Outport  Port=2  VectorParamsAs1DForOutWhenUnconnected=off
  P33 : Outport  Port=3  VectorParamsAs1DForOutWhenUnconnected=off
  P51 : Outport  Port=4  VectorParamsAs1DForOutWhenUnconnected=off
  dP2_ex : Outport  Port=5  VectorParamsAs1DForOutWhenUnconnected=off
  dP2_in : Outport  Port=6  VectorParamsAs1DForOutWhenUnconnected=off
  T31 : Outport  Port=7  VectorParamsAs1DForOutWhenUnconnected=off
  T32 : Outport  Port=8  VectorParamsAs1DForOutWhenUnconnected=off
  T33 : Outport  Port=9  VectorParamsAs1DForOutWhenUnconnected=off
  T51 : Outport  Port=10  VectorParamsAs1DForOutWhenUnconnected=off
  Q2_11 : Outport  Port=11  VectorParamsAs1DForOutWhenUnconnected=off
  Q2_12 : Outport  Port=12  VectorParamsAs1DForOutWhenUnconnected=off
  Q2_51 : Outport  Port=13  VectorParamsAs1DForOutWhenUnconnected=off
  C1 : Outport  Port=14  VectorParamsAs1DForOutWhenUnconnected=off
  L_11 : Outport  Port=15  VectorParamsAs1DForOutWhenUnconnected=off
  L_12 : Outport  Port=16  VectorParamsAs1DForOutWhenUnconnected=off
  L_21 : Outport  Port=17  VectorParamsAs1DForOutWhenUnconnected=off
  L_22 : Outport  Port=18  VectorParamsAs1DForOutWhenUnconnected=off
  wires:
  Demux4/1 -> Q2_11/1
  Demux/2 -> Demux2/1
  Demux/4 -> Demux4/1
  Demux2/1 -> dP2_ex/1
  Demux/3 -> Demux3/1
  Demux/6 -> Demux6/1
  Demux/1 -> Demux1/1
  Demux3/4 -> T51/1
  Demux1/4 -> P51/1
  Demux3/2 -> T32/1
  Modbus Read/1 -> Demux/1
  Demux6/1 -> L_11/1
  Demux6/2 -> L_12/1
  Demux4/3 -> Q2_51/1
  Demux4/2 -> Q2_12/1
  Demux6/3 -> L_21/1
  Demux6/4 -> L_22/1
  Demux3/3 -> T33/1
  Demux1/1 -> P31/1
  Demux1/2 -> P32/1
  Demux/5 -> C1/1
  Demux1/3 -> P33/1
  Demux2/2 -> dP2_in/1
  Demux3/1 -> T31/1
  Mux/1 -> Modbus Write/1
  Mux1/1 -> Mux/1
  V_31/1 -> Mux1/1
  V_51/1 -> Mux1/2
  V_61/1 -> Mux1/3
  V_71/1 -> Mux1/4
  Pu_4/1 -> Mux2/4
  Pu_3/1 -> Mux2/3
  Pu_1/1 -> Mux2/1
  Pu_2/1 -> Mux2/2
  Mux2/1 -> Mux/2
  Pu_5/1 -> Mux2/5
  Pu_6/1 -> Mux2/6
  Data/1 -> Mux/3
  Constant/1 -> Mux/4

== matlab function MPC_simulink/Auxillary Control/Auxillary control ==
  settings: updateMethod=DISCRETE  sampleTime=1
  data: dp input; pumpsaux output; u_aux input
function pumpsaux = controller(dp,u_aux)

persistent pumpctrlaux;        %Create persistent such that previous value of controller can be stored

if isempty(pumpctrlaux)
    pumpctrlaux=0;
end


if dp>0.45                   %Set high limit of level
    pumpsaux=u_aux;                    %Stop the pumps if level goes above 'high level' (in mm)
elseif dp<0.35                  %Set low limit of level
    pumpsaux=0;                  %Start the pumps if level goes below 'low level' (in mm)
else
    pumpsaux=pumpctrlaux;         %Run pump as the previous control command
    
end
pumpctrlaux=pumpsaux;             %Update persistent variable
end

== matlab function MPC_simulink/Auxillary Control/Auxillary control1 ==
  settings: updateMethod=DISCRETE
  data: dp input; pumpsaux output; u_aux input
function pumpsaux = controller(dp,u_aux)

persistent pumpctrlaux;        %Create persistent such that previous value of controller can be stored

if isempty(pumpctrlaux)
    pumpctrlaux=0;
end


if dp>0.45                       %Set high limit of level
    pumpsaux=u_aux;                    %Stop the pumps if level goes above 'high level' (in mm)
elseif dp<0.35                   %Set low limit of level
    pumpsaux=0;                  %Start the pumps if level goes below 'low level' (in mm)
else
    pumpsaux=pumpctrlaux;         %Run pump as the previous control command
    
end
pumpctrlaux=pumpsaux;             %Update persistent variable
end

== matlab function MPC_simulink/MATLAB Function ==
  data: trigger input; y output
function y = fcn(trigger)

persistent i_num

if isempty(i_num)
    i_num=0;
end

if trigger==1
    i_num=0;
end

i_num_v=i_num+1;

i_num=i_num_v;

y = i_num_v;
